simulink library "env2p_eng_std_std"  (Simulink 8.7)
settings: Solver=ode45  StartTime=0.0  StopTime=10.0  RelTol=1e-3
settings Model: Creator=rafrey5  LastModifiedBy=hillenb

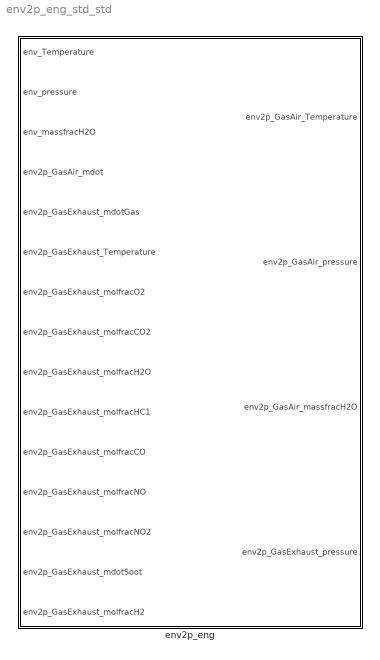
== system env2p_eng_std_std ==
  env2p_eng : Subsystem

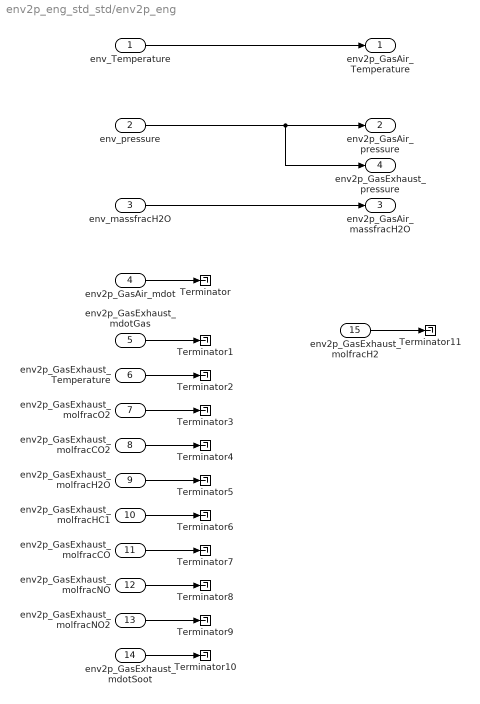
== system env2p_eng_std_std/env2p_eng ==
  env_Temperature : Inport
  env_pressure : Inport  Port=2
  env_massfracH2O : Inport  Port=3
  env2p_GasAir_mdot : Inport  Port=4
  env2p_GasExhaust_mdotGas : Inport  Port=5
  env2p_GasExhaust_Temperature : Inport  Port=6
  env2p_GasExhaust_molfracO2 : Inport  Port=7
  env2p_GasExhaust_molfracCO2 : Inport  Port=8
  env2p_GasExhaust_molfracH2O : Inport  Port=9
  env2p_GasExhaust_molfracHC1 : Inport  Port=10
  env2p_GasExhaust_molfracCO : Inport  Port=11
  env2p_GasExhaust_molfracNO : Inport  Port=12
  env2p_GasExhaust_molfracNO2 : Inport  Port=13
  env2p_GasExhaust_mdotSoot : Inport  Port=14
  env2p_GasExhaust_molfracH2 : Inport  Port=15
  Terminator{,1..11} (12 alike) : Terminator
  env2p_GasAir_Temperature : Outport
  env2p_GasAir_pressure : Outport  Port=2
  env2p_GasAir_massfracH2O : Outport  Port=3
  env2p_GasExhaust_pressure : Outport  Port=4
  wires:
  env2p_GasExhaust_mdotSoot/1 -> Terminator10/1
  env2p_GasExhaust_molfracNO2/1 -> Terminator9/1
  env2p_GasExhaust_molfracNO/1 -> Terminator8/1
  env2p_GasExhaust_molfracCO/1 -> Terminator7/1
  env2p_GasExhaust_molfracHC1/1 -> Terminator6/1
  env2p_GasExhaust_molfracH2O/1 -> Terminator5/1
  env2p_GasExhaust_molfracCO2/1 -> Terminator4/1
  env2p_GasExhaust_molfracO2/1 -> Terminator3/1
  env2p_GasExhaust_Temperature/1 -> Terminator2/1
  env2p_GasExhaust_mdotGas/1 -> Terminator1/1
  env2p_GasAir_mdot/1 -> Terminator/1
  env_massfracH2O/1 -> env2p_GasAir_massfracH2O/1
  env_pressure/1 -> env2p_GasExhaust_pressure/1, env2p_GasAir_pressure/1
  env_Temperature/1 -> env2p_GasAir_Temperature/1
  env2p_GasExhaust_molfracH2/1 -> Terminator11/1
